simulink model "Kinematics"  (R2020a)
settings: Solver=ode45  StartTime=0.0  StopTime=50  MaxStep=1e-4  MinStep=1e-6  RelTol=1e-3
settings Model: PacingRate=1.300000  Creator=gucos  LastModifiedBy=gucos
settings SolverCC: InitialStep=1e-6

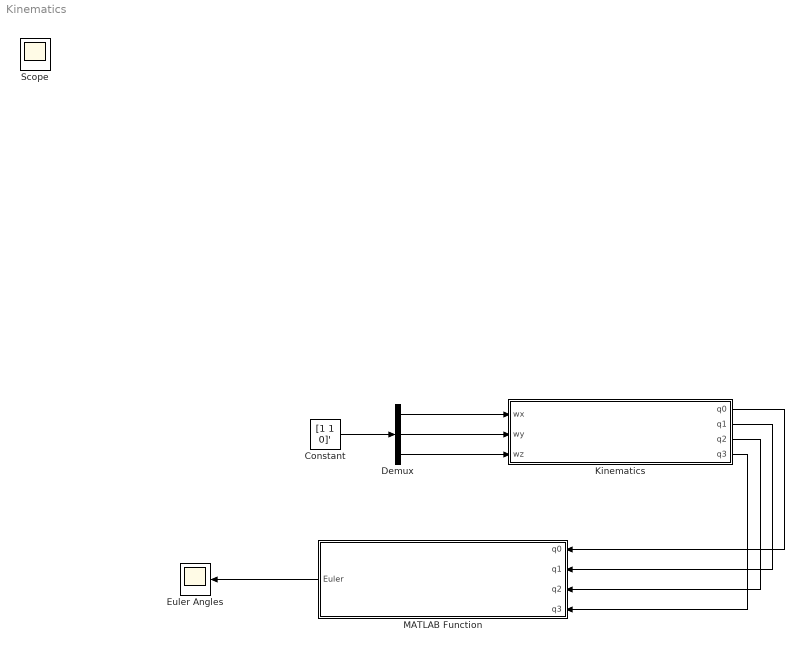
== system Kinematics ==
  Constant : Constant  Value=[1 1 0]'
  Demux : Demux  Outputs=3
  Euler Angles : Scope
  Kinematics : Subsystem
  MATLAB Function : MATLAB Function  TreatAsAtomicUnit=on
  Scope : Scope
  wires:
  MATLAB Function/1(Euler) -> Euler Angles/1
  Kinematics/1(q0) -> MATLAB Function/1(q0)
  Kinematics/2(q1) -> MATLAB Function/2(q1)
  Kinematics/3(q2) -> MATLAB Function/3(q2)
  Kinematics/4(q3) -> MATLAB Function/4(q3)
  Demux/1 -> Kinematics/1(wx)
  Demux/2 -> Kinematics/2(wy)
  Demux/3 -> Kinematics/3(wz)
  Constant/1 -> Demux/1

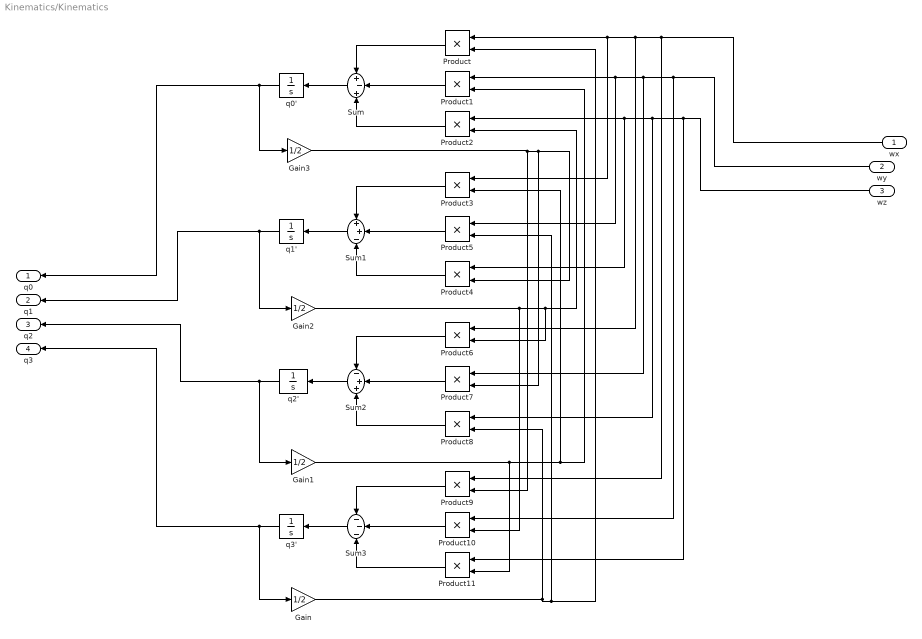
== system Kinematics/Kinematics ==
  wx : Inport
  wy : Inport  Port=2
  wz : Inport  Port=3
  Gain{,1..3} (4 alike) : Gain  Gain=1/2
  Product{,1..11} (12 alike) : Product
  Sum : Sum  Inputs=+-+
  Sum1 : Sum  Inputs=++-
  Sum2 : Sum  Inputs=-++
  Sum3 : Sum  Inputs=---
  q0' : Integrator  InitialCondition=-1
  q1' : Integrator
  q2' : Integrator
  q3' : Integrator
  q0 : Outport
  q1 : Outport  Port=2
  q2 : Outport  Port=3
  q3 : Outport  Port=4
  wires:
  Product10/1 -> Sum3/2
  wx/1 -> Product9/1, Product6/1, Product3/1, Product/1
  Gain/1 -> Product5/2, Product/2, Product8/2
  Product9/1 -> Sum3/1
  q2'/1 -> q2/1, Gain1/1
  Product11/1 -> Sum3/3
  wz/1 -> Product11/1, Product8/1, Product4/1, Product2/1
  q3'/1 -> q3/1, Gain/1
  Gain1/1 -> Product11/2, Product3/2, Product1/2
  Product1/1 -> Sum/2
  Product/1 -> Sum/1
  Gain3/1 -> Product9/2, Product7/2, Product4/2
  Sum/1 -> q0'/1
  Product6/1 -> Sum2/1
  Gain2/1 -> Product10/2, Product6/2, Product2/2
  Product7/1 -> Sum2/2
  q1'/1 -> q1/1, Gain2/1
  wy/1 -> Product10/1, Product7/1, Product5/1, Product1/1
  Sum1/1 -> q1'/1
  Product3/1 -> Sum1/1
  Product2/1 -> Sum/3
  Sum3/1 -> q3'/1
  q0'/1 -> Gain3/1, q0/1
  Product5/1 -> Sum1/2
  Sum2/1 -> q2'/1
  Product4/1 -> Sum1/3
  Product8/1 -> Sum2/3

== matlab function Kinematics/MATLAB Function ==
  data: q0 input; Euler output; q1 input; q2 input; q3 input

function Euler = ZYX(q0, q1, q2, q3)


C11 = (q0^2)+(q1^2)-(q2^2)-(q3^2);
C12 = (2*(q1*q2+q0*q3));
C13 = (2*(q1*q3-q0*q2));
%C21 = 2*(q1*q2-q0*q3)
%C22 = (q0^2)-(q1^2)+(q2^2)-(q3^2)
C23 = (2*(q2*q3+q0*q1));
%C31 = 2*(q1*q3+q0*q2)
%C32 = 2*(q2*q3-q0*q1)
C33 = ((q0^2)-(q1^2)-(q2^2)+(q3^2));

%C = [C11 C12 C13; C21 C22 C23; C31 C32 C33]

%DCM = [ctheta*calpha ctheta*salpha -stheta; sphi*stheta*calpha-cphi*salpha
%sphi*stheta*salpha+cphi*calpha sphi*ctheta; cphi*stheta*calpha+sphi*salpha
%cphi*stheta*salpha-sphi*calpha cphi*calpha]

theta = asind(-C13);


if C12 >= 0 && C11 >= 0
    
    if C23 >= 0 && C33 >= 0

        alpha = atand(C12/C11);
        phi = atand(C23/C33);

    elseif C23 >= 0 && C33 <= 0 

        alpha = atand(C12/C11);
        phi = atand(C23/C33) + 180;
        
    elseif C23 <= 0 && C33 <= 0

         alpha = atand(C12/C11);
         phi = atand(C23/C33) - 180;

    elseif C23 <= 0 && C33 >= 0

        alpha = atand(C12/C11);
        phi = atand(C23/C33);
        
         
    else
        
        alpha = 0;
        phi = 0;


    end

    
elseif C12 >= 0 && C11 <= 0 
    
    if C23 >= 0 && C33 >= 0

        alpha = atand(C12/C11) + 180;
        phi = atand(C23/C33);

    elseif C23 >= 0 && C33 <= 0 

        if q1 == 0 && q3 == 0
            alpha = atand(C12/C11);
            phi = atand(C23/C33);
        else
            alpha = atand(C12/C11) + 180;
            phi = atand(C23/C33) + 180;
        end
        
    elseif C23 <= 0 && C33 <= 0

         alpha = atand(C12/C11) + 180;
         phi = atand(C23/C33) - 180;

    elseif C23 <= 0 && C33 >= 0

        alpha = atand(C12/C11) + 180;
        phi = atand(C23/C33);
        
         
    else
        
        alpha = 0;
        phi = 0;


    end
    
    
elseif C12 <= 0 && C11 <= 0
    
    if C23 >= 0 && C33 >= 0

        alpha = atand(C12/C11) - 180;
        phi = atand(C23/C33);

    elseif C23 >= 0 && C33 <= 0 

        alpha = atand(C12/C11) - 180;
        phi = atand(C23/C33) + 180;
        
    elseif C23 <= 0 && C33 <= 0

         alpha = atand(C12/C11) - 180;
         phi = atand(C23/C33) - 180;

    elseif C23 <= 0 && C33 >= 0

        alpha = atand(C12/C11) - 180;
        phi = atand(C23/C33);
        
         
    else
        
        alpha = 0;
        phi = 0;


    end
     
     
elseif C12 <= 0 && C11 >= 0
    
    if C23 >= 0 && C33 >= 0

        alpha = atand(C12/C11);
        phi = atand(C23/C33);

    elseif C23 >= 0 && C33 <= 0 

        alpha = atand(C12/C11);
        phi = atand(C23/C33) + 180;
        
    elseif C23 <= 0 && C33 <= 0

         alpha = atand(C12/C11);
         phi = atand(C23/C33) - 180;

    elseif C23 <= 0 && C33 >= 0

        alpha = atand(C12/C11);
        phi = atand(C23/C33);
        
    else
        
        alpha = 0;
        phi = 0;

    end
    
else
    
    alpha = 0;
    phi = 0;
    
end

Euler = [alpha theta phi];
end
